simulink model "untitled_D2"  (R2013b)
settings: Solver=ode45  StartTime=0.0  StopTime=500  RelTol=1e-3
undefined symbols (not defined in the file): c, delta, kd, Qs, R
settings Model: Creator=Yurii  LastModifiedBy=Yurii

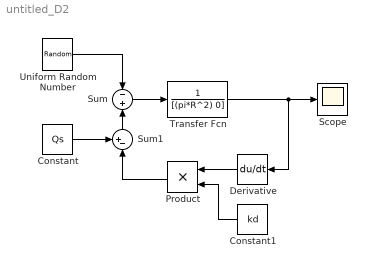
== system untitled_D2 ==
  Constant : Constant  Value=Qs
  Constant1 : Constant  Value=kd
  Derivative : Derivative
  Product : Product
  Scope : Scope
  Sum : Sum  Inputs=-|+
  Sum1 : Sum  Inputs=+-|
  Transfer Fcn : TransferFcn  Denominator=[(pi*R^2) 0]
  Uniform Random Number : UniformRandomNumber  Minimum=(c-delta)*Qs  Maximum=(c+delta)*Qs  SampleTime=0.1
  wires:
  Uniform Random Number/1 -> Sum/1
  Sum/1 -> Transfer Fcn/1
  Transfer Fcn/1 -> Derivative/1, Scope/1
  Constant1/1 -> Product/2
  Constant/1 -> Sum1/1
  Sum1/1 -> Sum/2
  Product/1 -> Sum1/2
  Derivative/1 -> Product/1
